simulink model "TestMotorSystem"  (R2018a)
settings: Solver=ode14x  StartTime=0.0  StopTime=10  FixedStep=Ts  RelTol=1e-3
values from neighbouring files (symbols this model uses):
  idrv = zeros(size(omegarv))    [setupTestMotorSystem.m]
  K_i = Omega_bw*R    (= 23)    [setupTestMotorSystem.m]
  K_p = Omega_bw*L    (= 0.1)    [setupTestMotorSystem.m]
  L_M = L    (= 0.001)    [setupTestMotorSystem.m]
  LamPM_M = Lambda_PM    (= 0.3)    [setupTestMotorSystem.m]
  NPoles_M = N_p    (= 6)    [setupTestMotorSystem.m]
  omegarv = linspace(0,800,1000)    [setupTestMotorSystem.m]
  Ts = 0.001    [setupTestMotorSystem.m]
undefined symbols (not defined in the file or in its folder): SJac_Per_I, Vdc_M
libraries: simulink_extras x3, simulink x2, Lib_PFSys_HiFiPMSM_TMATS x1
settings Model: Creator=glthoma1  LastModifiedBy=mebell
settings CodeAppCC: StateflowObjectComments=on

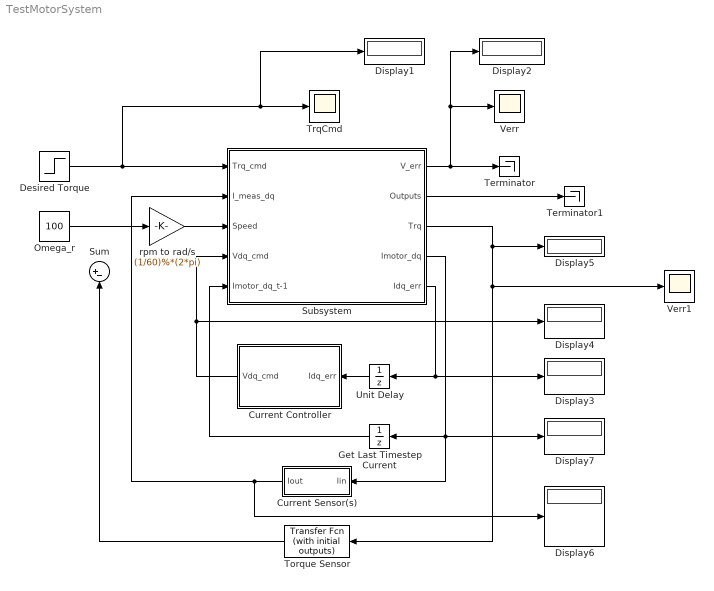
== system TestMotorSystem ==
  Current Controller : Subsystem
  Current Sensor(s) : Subsystem
  Desired Torque : Step  Time=5  Before=450  After=0  SampleTime=0
  Display{1..7} (7 alike) : Display
  Get Last Timestep Current : UnitDelay  InitialCondition=[-300; 330]  SampleTime=-1
  Omega_r : Constant  Value=100
  Subsystem : Subsystem
  Sum : Sum  Inputs=|+-
  Terminator : Terminator
  Terminator1 : Terminator
  Torque Sensor : simulink_extras/Additional Linear/Transfer Fcn (with initial outputs)  N=[10]  D="[1  10]"  Y0=450  U0=450
  TrqCmd : Scope
  Unit Delay : UnitDelay  InitialCondition=[0; 0]  SampleTime=-1
  Verr : Scope
  Verr1 : Scope
  rpm to rad/s : Gain  Gain=(1/60)%*(2*pi)
  wires:
  Desired Torque/1 -> Subsystem/1(Trq_cmd), Display1/1, TrqCmd/1
  Torque Sensor/1 -> Sum/2
  Subsystem/1(V_err) -> Terminator/1, Verr/1, Display2/1
  Current Sensor(s)/1(Iout) -> Display6/1, Subsystem/2(I_meas_dq)
  Omega_r/1 -> rpm to rad/s/1
  Subsystem/2(Outputs) -> Terminator1/1
  Subsystem/3(Trq) -> Verr1/1, Torque Sensor/1, Display5/1
  Subsystem/4(Imotor_dq) -> Current Sensor(s)/1(Iin), Display7/1, Get Last Timestep Current/1
  Subsystem/5(Idq_err) -> Display3/1, Unit Delay/1
  Current Controller/1(Vdq_cmd) -> Display4/1, Subsystem/4(Vdq_cmd)
  Unit Delay/1 -> Current Controller/1(Idq_err)
  rpm to rad/s/1 -> Subsystem/3(Speed)
  Get Last Timestep Current/1 -> Subsystem/5(Imotor_dq_t-1)

== system TestMotorSystem/Current Controller ==
  Idq_err : Inport
  Demux : Demux  Outputs=2
  Direct PID Controller : simulink/Continuous/PID Controller  Controller=PID  TimeDomain=Continuous-time  SampleTime=-1  IntegratorMethod=Forward Euler  FilterMethod=Forward Euler  Form=Parallel  UseFilter=on  ControllerParametersSource=internal  P=K_p  I=K_i  D=0  N=100  InitialConditionSource=internal  InitialConditionForIntegrator=-165  InitialConditionForFilter=0  ExternalReset=none  LimitOutput=off  UpperSaturationLimit=inf  LowerSaturationLimit=-inf  LinearizeAsGain=on  AntiWindupMode=none  Kb=1  TrackingMode=off  Kt=1  PParamMin=[]  PParamMax=[]  IParamMin=[]  IParamMax=[]  DParamMin=[]  DParamMax=[]  NParamMin=[]  NParamMax=[]  KbParamMin=[]  KbParamMax=[]  KtParamMin=[]  KtParamMax=[]  POutMin=[]  POutMax=[]  IOutMin=[]  IOutMax=[]  DOutMin=[]  DOutMax=[]  NOutMin=[]  NOutMax=[]  KbOutMin=[]  KbOutMax=[]  KtOutMin=[]  KtOutMax=[]  IntegratorOutMin=[]  IntegratorOutMax=[]  FilterOutMin=[]  FilterOutMax=[]  SumOutMin=[]  SumOutMax=[]  SumI1OutMin=[]  SumI1OutMax=[]  SumI2OutMin=[]  SumI2OutMax=[]  SumI3OutMin=[]  SumI3OutMax=[]  SumDOutMin=[]  SumDOutMax=[]  SaturationOutMin=[]  SaturationOutMax=[]  IntegratorContinuousStateAttributes=''  IntegratorStateMustResolveToSignalObject=off  IntegratorRTWStateStorageClass=Auto  FilterContinuousStateAttributes=''  FilterStateMustResolveToSignalObject=off  FilterRTWStateStorageClass=Auto  DifferentiatorICPrevScaledInput=0  DifferentiatorOutMin=[]  DifferentiatorOutMax=[]  InitialConditionSetting=State (most efficient)  FilterDiffOutCoefMin=[]  FilterDiffOutCoefMax=[]  SumDenOutMin=[]  SumDenOutMax=[]  SumNumOutMin=[]  SumNumOutMax=[]  ReciprocalOutMin=[]  ReciprocalOutMax=[]  DivideOutMin=[]  DivideOutMax=[]  TunerSelectOption=Transfer Function Based (PID Tuner App)
  Mux : Mux  Inputs=2
  Quadrature PID Controller : simulink/Continuous/PID Controller  Controller=PID  TimeDomain=Continuous-time  SampleTime=-1  IntegratorMethod=Forward Euler  FilterMethod=Forward Euler  Form=Parallel  UseFilter=on  ControllerParametersSource=internal  P=K_p  I=K_i  D=0  N=100  InitialConditionSource=internal  InitialConditionForIntegrator=76  InitialConditionForFilter=0  ExternalReset=none  LimitOutput=off  UpperSaturationLimit=inf  LowerSaturationLimit=-inf  LinearizeAsGain=on  AntiWindupMode=none  Kb=1  TrackingMode=off  Kt=1  PParamMin=[]  PParamMax=[]  IParamMin=[]  IParamMax=[]  DParamMin=[]  DParamMax=[]  NParamMin=[]  NParamMax=[]  KbParamMin=[]  KbParamMax=[]  KtParamMin=[]  KtParamMax=[]  POutMin=[]  POutMax=[]  IOutMin=[]  IOutMax=[]  DOutMin=[]  DOutMax=[]  NOutMin=[]  NOutMax=[]  KbOutMin=[]  KbOutMax=[]  KtOutMin=[]  KtOutMax=[]  IntegratorOutMin=[]  IntegratorOutMax=[]  FilterOutMin=[]  FilterOutMax=[]  SumOutMin=[]  SumOutMax=[]  SumI1OutMin=[]  SumI1OutMax=[]  SumI2OutMin=[]  SumI2OutMax=[]  SumI3OutMin=[]  SumI3OutMax=[]  SumDOutMin=[]  SumDOutMax=[]  SaturationOutMin=[]  SaturationOutMax=[]  IntegratorContinuousStateAttributes=''  IntegratorStateMustResolveToSignalObject=off  IntegratorRTWStateStorageClass=Auto  FilterContinuousStateAttributes=''  FilterStateMustResolveToSignalObject=off  FilterRTWStateStorageClass=Auto  DifferentiatorICPrevScaledInput=0  DifferentiatorOutMin=[]  DifferentiatorOutMax=[]  InitialConditionSetting=State (most efficient)  FilterDiffOutCoefMin=[]  FilterDiffOutCoefMax=[]  SumDenOutMin=[]  SumDenOutMax=[]  SumNumOutMin=[]  SumNumOutMax=[]  ReciprocalOutMin=[]  ReciprocalOutMax=[]  DivideOutMin=[]  DivideOutMax=[]  TunerSelectOption=Transfer Function Based (PID Tuner App)
  Vdq_cmd : Outport
  wires:
  Demux/2 -> Quadrature PID Controller/1
  Demux/1 -> Direct PID Controller/1
  Direct PID Controller/1 -> Mux/1
  Quadrature PID Controller/1 -> Mux/2
  Idq_err/1 -> Demux/1
  Mux/1 -> Vdq_cmd/1

== system TestMotorSystem/Current Sensor(s) ==
  Iin : Inport
  Current Sensor : simulink_extras/Additional Linear/Transfer Fcn (with initial outputs)  N=[10000]  D="[1  10000]"  Y0=-300  U0=-300
  Current Sensor1 : simulink_extras/Additional Linear/Transfer Fcn (with initial outputs)  N=[10000]  D="[1  10000]"  Y0=330  U0=330
  Demux : Demux  Outputs=2
  Mux : Mux  Inputs=2
  Iout : Outport
  wires:
  Iin/1 -> Demux/1
  Demux/1 -> Current Sensor/1
  Demux/2 -> Current Sensor1/1
  Current Sensor/1 -> Mux/1
  Current Sensor1/1 -> Mux/2
  Mux/1 -> Iout/1

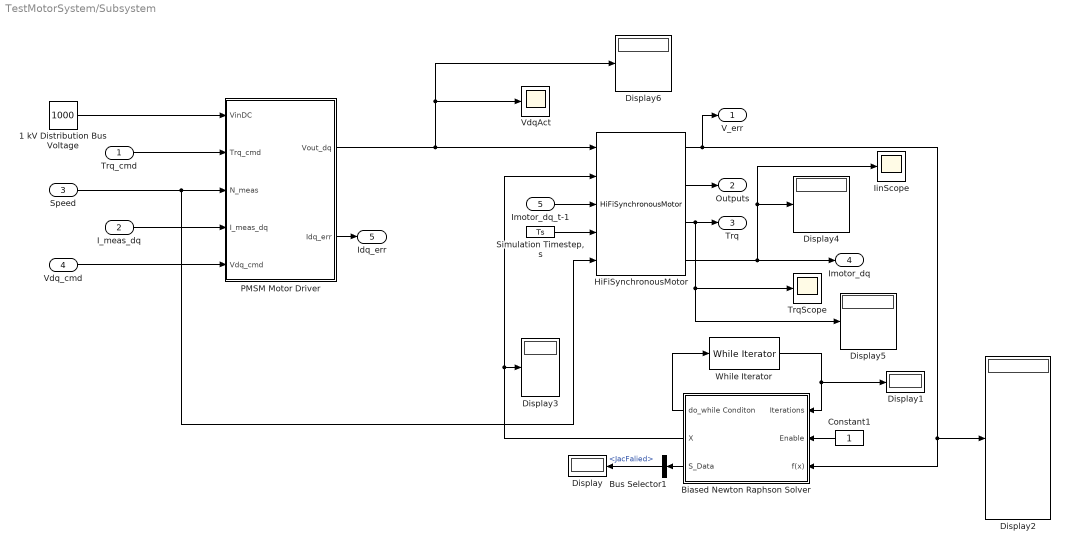
== system TestMotorSystem/Subsystem ==
  Trq_cmd : Inport
  I_meas_dq : Inport  Port=2
  Speed : Inport  Port=3
  Vdq_cmd : Inport  Port=4
  Imotor_dq_t-1 : Inport  Port=5
  1 kV Distribution Bus Voltage : Constant  Value=1000
  Biased Newton Raphson Solver : Subsystem  mask(Newton Raphson Solver){SJac_Per_M=0.001*[1; -1]*([1 1]), SNR_IC_M=[-300; 330], Shift_M=1000, SNR_DX_M=0.5, SNR_Mx_M=1e5, SNR_Mn_M=-1e5, SJacobianAttempts_M=2, Cond_Limits_M=0.001}
      mask prompts: SJac_Per_M "SJac_Per_M - Jacobian Perturbation size (frac) (nxm)"; SNR_IC_M "SNR_IC_M - Newton Raphson Initial Conditions (mx1)"; Shift_M "Shift_M - Bias to shift the solution to avoid convergence issues"; SNR_DX_M "SNR_DX_M - Newton Raphson step size limiter (%) (1x1)"; SNR_Mx_M "SNR_Mx_M - Newton Raphson max limit (1x1 or mx1)"; SNR_Mn_M "SNR_Mn_M - Newton Raphson min limit (1x1 or mx1)"; SJacobianAttempts_M "SJacobianAttempts_M - Newton Raphson attempts before the Jacobian recalculation (1x1)"; Cond_Limits_M "Cond_Limits_M - Iteration Conditions Limits (mx1 or 1x1)"
      mask help:
      | The Iterative Newton Raphson Solver with Jacobian Calculator block will
      | supply the inputs to iteratively drive the outputs of a system to zero.
      |
      | This will be performed in three steps.
      | 1) Jabobian calculator sends Perturbations to the plant then calculates the plant
      | Jacboian based on the system response
      | 2) The Newton Raphson will use the inverse of the Jacobian to iteratively step the
      | system toward solution.
      | 3) Once the solution has satisfied the conditions the Newton Raphson is shut off.
      |
      | This module is designed for dynamic systems and should be paired with
      | a "do... while" block in Simulink. The "do...while" block and this module
      | should both be located in the same subsystem as the plant that is to be solved for.
      mask init:
      | if isequal(size(SNR_Mx_M),size(SNR_IC_M))
      | elseif isequal(size(SNR_Mx_M),[1 1])
      | else
      |     disp('NR_Mx_Lim_M must be the same size as NR_IC_M or a constant')
      | end
      | 
      | if isequal(size(SNR_Mn_M),size(SNR_IC_M))
      | elseif isequal(size(SNR_Mn_M),[1 1])
      | else
      |     disp('NR_Mn_Lim_M must be the same size as NR_IC_M or a constant')
      | end
      | 
      | for i = 1:size(SJac_Per_M,1)
      |     SJac_Per_I(i,:) = SJac_Per_M(i,:).*(SNR_IC_M'./(SNR_IC_M' + Shift_M));
      | end
      mask Help: web(which('Solver_TMATS_INRSwJC.html'),'-helpbrowser')
  Bus Selector1 : BusSelector  OutputSignals=JacFalied
  Constant1 : Constant
  Display{,1..6} (7 alike) : Display
  HiFiSynchronousMotor : Lib_PFSys_HiFiPMSM_TMATS/HiFiSynchronousMotor  X_C_TorqueVec_M=[0 1000 10000]  Y_C_SpeedVec_M=[0 500 5000]  T_C_EffArray_M=[0.5 0.5 0.5; 0.5 1 1; 0.5 1 1]  R_M=R  L_M=L  LamPM_M=Lambda_PM  NPoles_M=N_p  NPhases_M=N_phases
  IinScope : Scope
  PMSM Motor Driver : Subsystem
  "Simulation Timestep, s" : Constant  Value=Ts
  TrqScope : Scope
  VdqAct : Scope
  While Iterator : WhileIterator  MaxIters=20  WhileBlockType=do-while  ShowIterationPort=on
  V_err : Outport
  Outputs : Outport  Port=2
  Trq : Outport  Port=3
  Imotor_dq : Outport  Port=4
  Idq_err : Outport  Port=5
  wires:
  HiFiSynchronousMotor/4 -> IinScope/1, Display4/1, Imotor_dq/1
  "Simulation Timestep, s"/1 -> HiFiSynchronousMotor/4
  Speed/1 -> HiFiSynchronousMotor/5, PMSM Motor Driver/3(N_meas)
  HiFiSynchronousMotor/2 -> Outputs/1
  Biased Newton Raphson Solver/2(X) -> HiFiSynchronousMotor/2, Display3/1
  Biased Newton Raphson Solver/3(S_Data) -> Bus Selector1/1
  HiFiSynchronousMotor/1 -> Display2/1, Biased Newton Raphson Solver/3(f(x)), V_err/1
  While Iterator/1 -> Biased Newton Raphson Solver/1(Iterations), Display1/1
  Biased Newton Raphson Solver/1(do_while Conditon) -> While Iterator/1
  Bus Selector1/1 -> Display/1  "<JacFalied>"
  Constant1/1 -> Biased Newton Raphson Solver/2(Enable)
  HiFiSynchronousMotor/3 -> TrqScope/1, Display5/1, Trq/1
  PMSM Motor Driver/1(Vout_dq) -> HiFiSynchronousMotor/1, Display6/1, VdqAct/1
  1 kV Distribution Bus Voltage/1 -> PMSM Motor Driver/1(VinDC)
  Trq_cmd/1 -> PMSM Motor Driver/2(Trq_cmd)
  I_meas_dq/1 -> PMSM Motor Driver/4(I_meas_dq)
  Vdq_cmd/1 -> PMSM Motor Driver/5(Vdq_cmd)
  PMSM Motor Driver/2(Idq_err) -> Idq_err/1
  Imotor_dq_t-1/1 -> HiFiSynchronousMotor/3

== system TestMotorSystem/Subsystem/Biased Newton Raphson Solver ==
  Iterations : Inport
  Enable : Inport  Port=2
  f(x) : Inport  Port=3
  Constant2 : Constant  Value=Shift_M
  Iterative NR Solver w JacobianCalc : Subsystem  mask(T-MATS: Iterative NR Solver w Jacobian Calc Library Block){SJac_Per_M=SJac_Per_I, SNR_IC_M=SNR_IC_M + Shift_M, SNR_DX_M=SNR_DX_M, SNR_Mx_M=SNR_Mx_M, SNR_Mn_M=SNR_Mn_M, SJacobianAttempts_M=SJacobianAttempts_M, Cond_Limits_M=Cond_Limits_M}
      mask prompts: SJac_Per_M "SJac_Per_M - Jacobian Perturbation size (frac) (nxm)"; SNR_IC_M "SNR_IC_M - Newton Raphson Initial Conditions (mx1)"; SNR_DX_M "SNR_DX_M - Newton Raphson step size limiter (%) (1x1)"; SNR_Mx_M "SNR_Mx_M - Newton Raphson max limit (1x1 or mx1)"; SNR_Mn_M "SNR_Mn_M - Newton Raphson min limit (1x1 or mx1)"; SJacobianAttempts_M "SJacobianAttempts_M - Newton Raphson attempts before the Jacobian recalculation (1x1)"; Cond_Limits_M "Cond_Limits_M - Iteration Conditions Limits (mx1 or 1x1)"
      mask help:
      | The Iterative Newton Raphson Solver with Jacobian Calculator block will
      | supply the inputs to iteratively drive the outputs of a system to zero.
      |
      | This will be performed in three steps.
      | 1) Jabobian calculator sends Perturbations to the plant then calculates the plant
      | Jacboian based on the system response
      | 2) The Newton Raphson will use the inverse of the Jacobian to iteratively step the
      | system toward solution.
      | 3) Once the solution has satisfied the conditions the Newton Raphson is shut off.
      |
      | This module is designed for dynamic systems and should be paired with
      | a "do... while" block in Simulink. The "do...while" block and this module
      | should both be located in the same subsystem as the plant that is to be solved for.
      mask init:
      | if isequal(size(SNR_Mx_M),size(SNR_IC_M))
      | elseif isequal(size(SNR_Mx_M),[1 1])
      | else
      |     disp('NR_Mx_Lim_M must be the same size as NR_IC_M or a constant')
      | end
      | 
      | if isequal(size(SNR_Mn_M),size(SNR_IC_M))
      | elseif isequal(size(SNR_Mn_M),[1 1])
      | else
      |     disp('NR_Mn_Lim_M must be the same size as NR_IC_M or a constant')
      | end
      mask Help: web(which('Solver_TMATS_INRSwJC.html'),'-helpbrowser')
  Sum : Sum  Inputs=|+-
  do_while Conditon : Outport
  X : Outport  Port=2
  S_Data : Outport  Port=3
  wires:
  Constant2/1 -> Sum/2
  Iterative NR Solver w JacobianCalc/2(X) -> Sum/1
  f(x)/1 -> Iterative NR Solver w JacobianCalc/3(f(x))
  Iterations/1 -> Iterative NR Solver w JacobianCalc/1(Iterations)
  Enable/1 -> Iterative NR Solver w JacobianCalc/2(Enable)
  Iterative NR Solver w JacobianCalc/3(S_Data) -> S_Data/1
  Iterative NR Solver w JacobianCalc/1(do_while Condition) -> do_while Conditon/1
  Sum/1 -> X/1

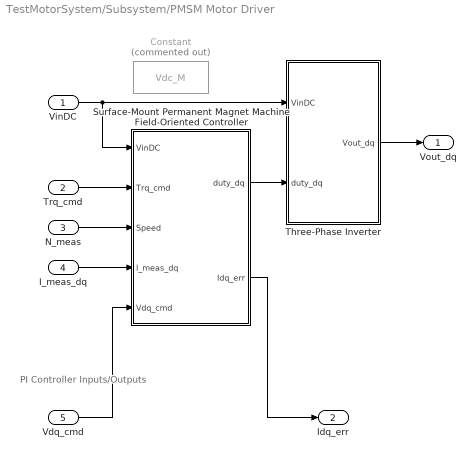
== system TestMotorSystem/Subsystem/PMSM Motor Driver ==
  note: PI Controller
      | Inputs/Outputs
  VinDC : Inport
  Trq_cmd : Inport  Port=2
  N_meas : Inport  Port=3
  I_meas_dq : Inport  Port=4
  Vdq_cmd : Inport  Port=5
  Constant : Constant  Commented=on  Value=Vdc_M
  Surface-Mount Permanent Magnet Machine Field-Oriented Controller : Subsystem
  Three-Phase Inverter : Subsystem
  Vout_dq : Outport
  Idq_err : Outport  Port=2
  wires:
  N_meas/1 -> Surface-Mount Permanent Magnet Machine Field-Oriented Controller/3(Speed)
  Surface-Mount Permanent Magnet Machine Field-Oriented Controller/1(duty_dq) -> Three-Phase Inverter/2(duty_dq)
  Trq_cmd/1 -> Surface-Mount Permanent Magnet Machine Field-Oriented Controller/2(Trq_cmd)
  I_meas_dq/1 -> Surface-Mount Permanent Magnet Machine Field-Oriented Controller/4(I_meas_dq)
  Three-Phase Inverter/1(Vout_dq) -> Vout_dq/1
  Surface-Mount Permanent Magnet Machine Field-Oriented Controller/2(Idq_err) -> Idq_err/1
  Vdq_cmd/1 -> Surface-Mount Permanent Magnet Machine Field-Oriented Controller/5(Vdq_cmd)
  VinDC/1 -> Surface-Mount Permanent Magnet Machine Field-Oriented Controller/1(VinDC), Three-Phase Inverter/1(VinDC)

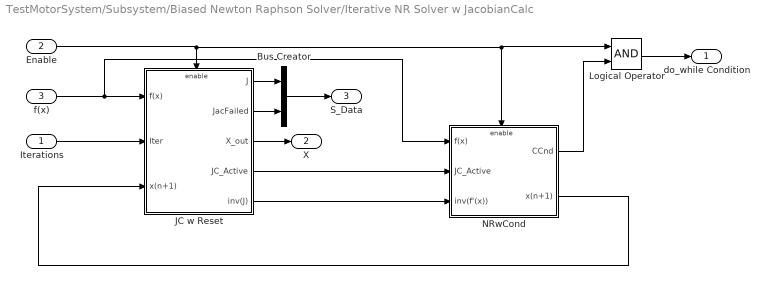
== system TestMotorSystem/Subsystem/Biased Newton Raphson Solver/Iterative NR Solver w JacobianCalc ==
  Iterations : Inport  PortDimensions=1
  Enable : Inport  Port=2  PortDimensions=1
  f(x) : Inport  Port=3  PortDimensions=length(SNR_IC_M)
  Bus Creator : BusCreator  Inputs=2
  JC w Reset : Subsystem
  Logical Operator : Logic  AllPortsSameDT=off  OutDataTypeStr=boolean
  NRwCond : Subsystem
  do_while Condition : Outport  PortDimensions=1
  X : Outport  Port=2  PortDimensions=length(SNR_IC_M)
  S_Data : Outport  Port=3
  wires:
  f(x)/1 -> NRwCond/1(f(x)), JC w Reset/1(f(x))
  NRwCond/1(CCnd) -> Logical Operator/2
  Iterations/1 -> JC w Reset/2(Iter)
  NRwCond/2(x(n+1)) -> JC w Reset/3(x(n+1))
  JC w Reset/1(J) -> Bus Creator/1
  JC w Reset/3(X_out) -> X/1
  JC w Reset/4(JC_Active) -> NRwCond/2(JC_Active)
  JC w Reset/5(inv(J)) -> NRwCond/3(inv(f'(x)))
  Enable/1 -> JC w Reset/Enable, NRwCond/Enable, Logical Operator/1
  Logical Operator/1 -> do_while Condition/1
  Bus Creator/1 -> S_Data/1
  JC w Reset/2(JacFailed) -> Bus Creator/2

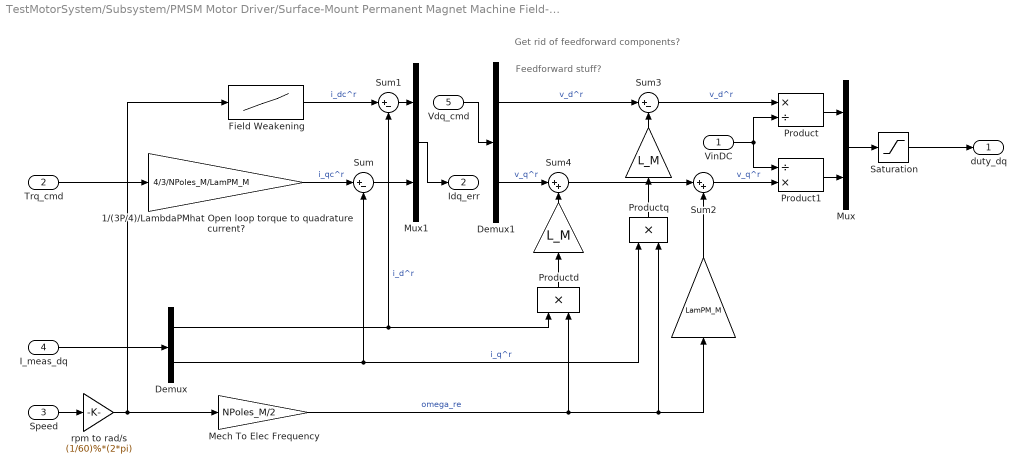
== system TestMotorSystem/Subsystem/PMSM Motor Driver/Surface-Mount Permanent Magnet Machine Field-Oriented Controller ==
  note: Feedforward stuff?
  note: Get rid of feedforward components?
  VinDC : Inport
  Trq_cmd : Inport  Port=2
  Speed : Inport  Port=3
  I_meas_dq : Inport  Port=4
  Vdq_cmd : Inport  Port=5
  "  " : Gain  Gain=L_M  SaturateOnIntegerOverflow=on  OutDataTypeStr=Inherit: Same as input  ParamDataTypeStr=Inherit: Same as input
  "   " : Gain  Gain=LamPM_M  SaturateOnIntegerOverflow=on  OutDataTypeStr=Inherit: Same as input  ParamDataTypeStr=Inherit: Same as input
  "      " : Gain  Gain=L_M  SaturateOnIntegerOverflow=on  OutDataTypeStr=Inherit: Same as input  ParamDataTypeStr=Inherit: Same as input
  1/(3P/4)/LambdaPMhat Open loop torque to quadrature current? : Gain  Gain=4/3/NPoles_M/LamPM_M  SaturateOnIntegerOverflow=on  OutDataTypeStr=Inherit: Same as input  ParamDataTypeStr=Inherit: Same as input
  Demux : Demux  Outputs=2
  Demux1 : Demux  Outputs=2
  Field Weakening : Lookup_n-D  NumberOfTableDimensions=1  BreakpointsForDimension1=omegarv  Table=idrv  InternalRulePriority=Speed  RndMeth=Simplest  InputSameDT=on
  Mech To Elec Frequency : Gain  Gain=NPoles_M/2  SaturateOnIntegerOverflow=on  OutDataTypeStr=Inherit: Same as input  ParamDataTypeStr=Inherit: Same as input
  Mux : Mux  Inputs=2
  Mux1 : Mux  Inputs=2
  Product : Product  Inputs=*/  SaturateOnIntegerOverflow=on  OutDataTypeStr=Inherit: Same as first input
  Product1 : Product  Inputs=/*  SaturateOnIntegerOverflow=on  OutDataTypeStr=Inherit: Same as first input
  Productd : Product  SaturateOnIntegerOverflow=on  OutDataTypeStr=Inherit: Same as first input
  Productq : Product  SaturateOnIntegerOverflow=on  OutDataTypeStr=Inherit: Same as first input
  Saturation : Saturate  UpperLimit=1  LowerLimit=0
  Sum : Sum  Inputs=|+-  SaturateOnIntegerOverflow=on
  Sum1 : Sum  Inputs=|+-  SaturateOnIntegerOverflow=on
  Sum2 : Sum  Inputs=|++  SaturateOnIntegerOverflow=on
  Sum3 : Sum  Inputs=|+-  SaturateOnIntegerOverflow=on
  Sum4 : Sum  Inputs=|++  SaturateOnIntegerOverflow=on
  rpm to rad/s : Gain  Gain=(1/60)%*(2*pi)
  duty_dq : Outport
  Idq_err : Outport  Port=2
  wires:
  Trq_cmd/1 -> 1/(3P/4)/LambdaPMhat Open loop torque to quadrature current?/1
  1/(3P/4)/LambdaPMhat Open loop torque to quadrature current?/1 -> Sum/1  "i_qc^r"
  Demux/1 -> Productd/1, Sum1/2  "i_d^r"
  Demux/2 -> Productq/1, Sum/2  "i_q^r"
  Field Weakening/1 -> Sum1/1  "i_dc^r"
  Sum1/1 -> Mux1/1
  Sum/1 -> Mux1/2
  Mech To Elec Frequency/1 -> "   "/1, Productq/2, Productd/2  "omega_re"
  Productq/1 -> "      "/1
  Sum3/1 -> Product/1  "v_d^r"
  "      "/1 -> Sum3/2
  "  "/1 -> Sum4/2
  Productd/1 -> "  "/1
  Demux1/2 -> Sum4/1  "v_q^r"
  Sum4/1 -> Sum2/1
  "   "/1 -> Sum2/2
  I_meas_dq/1 -> Demux/1
  Vdq_cmd/1 -> Demux1/1
  Mux1/1 -> Idq_err/1
  Demux1/1 -> Sum3/1  "v_d^r"
  Sum2/1 -> Product1/2  "v_q^r"
  VinDC/1 -> Product/2, Product1/1
  Product/1 -> Mux/1
  Product1/1 -> Mux/2
  Mux/1 -> Saturation/1
  Speed/1 -> rpm to rad/s/1
  rpm to rad/s/1 -> Mech To Elec Frequency/1, Field Weakening/1
  Saturation/1 -> duty_dq/1

== system TestMotorSystem/Subsystem/PMSM Motor Driver/Three-Phase Inverter ==
  VinDC : Inport
  duty_dq : Inport  Port=2
  Product : Product
  Vout_dq : Outport
  wires:
  duty_dq/1 -> Product/2
  VinDC/1 -> Product/1
  Product/1 -> Vout_dq/1

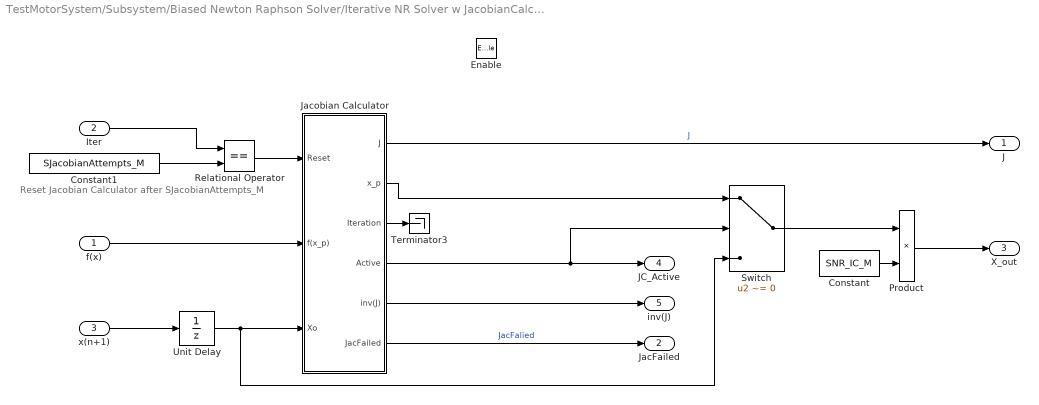
== system TestMotorSystem/Subsystem/Biased Newton Raphson Solver/Iterative NR Solver w JacobianCalc/JC w Reset ==
  note: Reset Jacobian Calculator after SJacobianAttempts_M
  f(x) : Inport  PortDimensions=length(SNR_IC_M)
  Iter : Inport  Port=2  PortDimensions=1
  x(n+1) : Inport  Port=3
  Enable : EnablePort
  Constant : Constant  Value=SNR_IC_M
  Constant1 : Constant  Value=SJacobianAttempts_M  OutDataTypeStr=uint32
  Jacobian Calculator : Subsystem  TreatAsAtomicUnit=on  mask(T-MATS: Jacobian Calculator Library Block){N_Per_M=SJac_Per_M}
      mask prompts: N_Per_M "N_Per_M - Perturbations (nxm)"
      mask help:
      | The Jacobian Calculator block calculates the Jabobian of the system by perturbing the system around an initial point and calculating the gradient for each perturbation. This module will run once on start up and then again only if the reset is pressed.
      | Below: n (rows) is the number of times each independent will be perturbed and m (columns) is the number of inputs.
      mask Help: web(which('NumMthd_TMATS_JC.html'),'-helpbrowser')
  Product : Product  RndMeth=Zero
  Relational Operator : RelationalOperator  Operator===  OutDataTypeStr=boolean  RndMeth=Nearest
  Switch : Switch  Criteria=u2 ~= 0  Threshold=1
  Terminator3 : Terminator
  Unit Delay : UnitDelay  InitialCondition=ones(length(SNR_IC_M),1)  SampleTime=-1
  J : Outport  PortDimensions=[length(SNR_IC_M),length(SNR_IC_M)]
  JacFailed : Outport  Port=2  PortDimensions=1
  X_out : Outport  Port=3  PortDimensions=length(SNR_IC_M)
  JC_Active : Outport  Port=4  PortDimensions=1
  inv(J) : Outport  Port=5  PortDimensions=[length(SNR_IC_M),length(SNR_IC_M)]
  wires:
  f(x)/1 -> Jacobian Calculator/2(f(x_p))
  Jacobian Calculator/5(inv(J)) -> inv(J)/1
  Unit Delay/1 -> Switch/3, Jacobian Calculator/3(Xo)
  x(n+1)/1 -> Unit Delay/1
  Jacobian Calculator/1(J) -> J/1  "J"
  Constant/1 -> Product/2
  Relational Operator/1 -> Jacobian Calculator/1(Reset)
  Product/1 -> X_out/1
  Jacobian Calculator/2(x_p) -> Switch/1
  Switch/1 -> Product/1
  Jacobian Calculator/4(Active) -> Switch/2, JC_Active/1
  Constant1/1 -> Relational Operator/2
  Iter/1 -> Relational Operator/1
  Jacobian Calculator/3(Iteration) -> Terminator3/1
  Jacobian Calculator/6(JacFailed) -> JacFailed/1  "JacFalied"

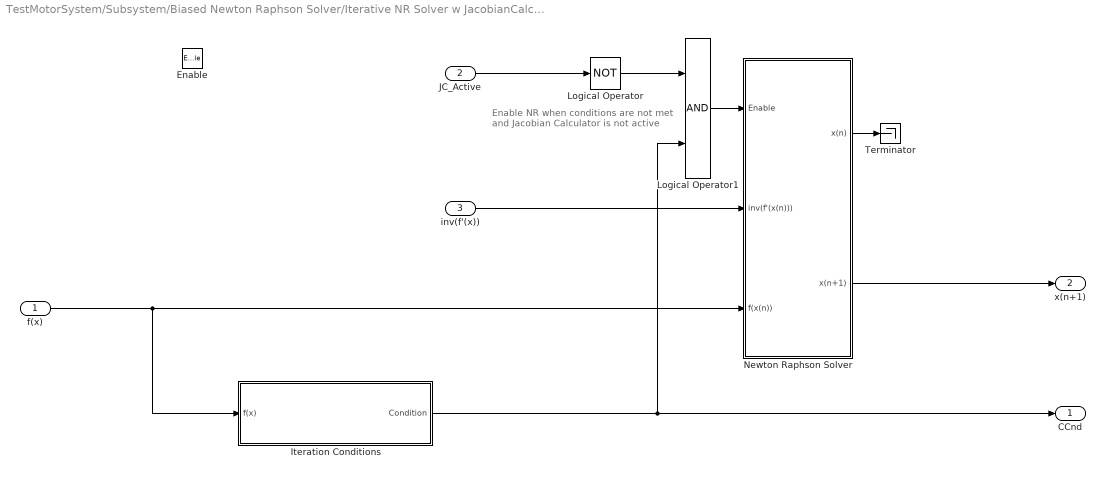
== system TestMotorSystem/Subsystem/Biased Newton Raphson Solver/Iterative NR Solver w JacobianCalc/NRwCond ==
  note: Enable NR when conditions are not met
      | and Jacobian Calculator is not active
  f(x) : Inport  PortDimensions=length(SNR_IC_M)
  JC_Active : Inport  Port=2  PortDimensions=1
  inv(f'(x)) : Inport  Port=3  PortDimensions=[length(SNR_IC_M),length(SNR_IC_M)]
  Enable : EnablePort
  Iteration Conditions : Subsystem
  Logical Operator : Logic  Operator=NOT  AllPortsSameDT=off  OutDataTypeStr=boolean
  Logical Operator1 : Logic  AllPortsSameDT=off  OutDataTypeStr=boolean
  Newton Raphson Solver : Subsystem  TreatAsAtomicUnit=on  mask(T-MATS: Newton Raphson Solver Library Block){NR_IC_M=ones(size(SNR_IC_M)), NR_dx_Lim_M=SNR_DX_M, NR_Mx_Lim_M=SNR_Mx_M./SNR_IC_M, NR_Mn_Lim_M=SNR_Mn_M./SNR_IC_M, BlkNm_M=double(gcb)}
      mask prompts: NR_IC_M "NR_IC_M - Initial Conditions of Newton Raphson (mx1)"; NR_dx_Lim_M "NR_dx_Lim_M - Newton Raphson step size limit (%) (1x1)"; NR_Mx_Lim_M "NR_Mx_Lim_M - Max limit (1x1 or mx1)"; NR_Mn_Lim_M "NR_Mn_Lim_M - Min Limit (1x1 or mx1)"; BlkNm_M "BlkNm_M - Block Name"
      mask help:
      | Newton Raphson Solver:
      |
      | x(n+1) = x(n) - inverse(f'(x(n)))*f(x(n))
      |
      | Note:
      | inverse(f'(x(n))) is an m x m matrix and f(x(n)) is an m x 1 matrix
      | where m is the length of the initial conditions matrix and number of system independents.
      mask init:
      | if isequal(size(NR_Mx_Lim_M),size(NR_IC_M))
      | elseif isequal(size(NR_Mx_Lim_M),size(1))
      | else
      |     warning('NR_Mx_Lim_M must be the same size as NR_IC_M or a constant')
      | end
      | 
      | if isequal(size(NR_Mn_Lim_M),size(NR_IC_M))
      | elseif isequal(size(NR_Mn_Lim_M),size(1))
      | else
      |     warning('NR_Mn_Lim_M must be the same size as NR_IC_M or a constant')
      | end
      mask Help: web(which('NumMthd_TMATS_NRS.html'),'-helpbrowser')
  Terminator : Terminator
  CCnd : Outport  PortDimensions=1
  x(n+1) : Outport  Port=2  PortDimensions=length(SNR_IC_M)
  wires:
  f(x)/1 -> Iteration Conditions/1(f(x)), Newton Raphson Solver/3(f(x(n)))
  JC_Active/1 -> Logical Operator/1
  Newton Raphson Solver/2(x(n+1)) -> x(n+1)/1
  Newton Raphson Solver/1(x(n)) -> Terminator/1
  inv(f'(x))/1 -> Newton Raphson Solver/2(inv(f'(x(n))))
  Logical Operator1/1 -> Newton Raphson Solver/1(Enable)
  Logical Operator/1 -> Logical Operator1/1
  Iteration Conditions/1(Condition) -> Logical Operator1/2, CCnd/1

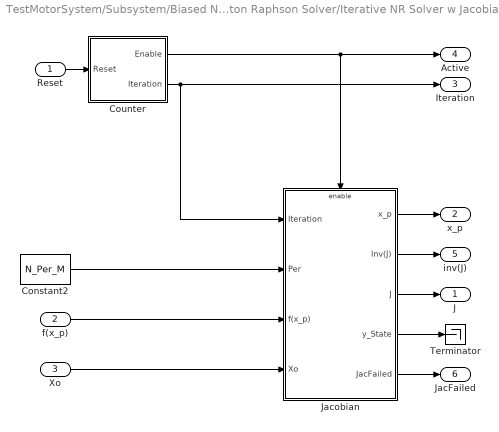
== system TestMotorSystem/Subsystem/Biased Newton Raphson Solver/Iterative NR Solver w JacobianCalc/JC w Reset/Jacobian Calculator ==
  Reset : Inport  PortDimensions=1
  f(x_p) : Inport  Port=2  PortDimensions=size(N_Per_M,2)
  Xo : Inport  Port=3  PortDimensions=size(N_Per_M,2)
  Constant2 : Constant  Value=N_Per_M
  Counter : Subsystem  mask{N_Ind_M=prod(size(N_Per_M))}
      mask prompts: N_Ind_M "number of independents, N_Ind_M"
  Jacobian : Subsystem
  Terminator : Terminator
  J : Outport  PortDimensions=[size(N_Per_M,2), size(N_Per_M,2)]
  x_p : Outport  Port=2  PortDimensions=size(N_Per_M,2)
  Iteration : Outport  Port=3  PortDimensions=1
  Active : Outport  Port=4  PortDimensions=1
  inv(J) : Outport  Port=5  PortDimensions=[size(N_Per_M,2), size(N_Per_M,2)]
  JacFailed : Outport  Port=6  PortDimensions=1
  wires:
  f(x_p)/1 -> Jacobian/3(f(x_p))
  Constant2/1 -> Jacobian/2(Per)
  Jacobian/1(x_p) -> x_p/1
  Reset/1 -> Counter/1(Reset)
  Counter/1(Enable) -> Active/1, Jacobian/Enable
  Xo/1 -> Jacobian/4(Xo)
  Counter/2(Iteration) -> Iteration/1, Jacobian/1(Iteration)
  Jacobian/2(Inv(J)) -> inv(J)/1
  Jacobian/3(J) -> J/1
  Jacobian/4(y_State) -> Terminator/1
  Jacobian/5(JacFailed) -> JacFailed/1

== system TestMotorSystem/Subsystem/Biased Newton Raphson Solver/Iterative NR Solver w JacobianCalc/NRwCond/Iteration Conditions ==
  f(x) : Inport
  Abs : Abs
  Constant1 : Constant  Value=Cond_Limits_M
  Constant2 : Constant  Value=0
  Relational Operator : RelationalOperator  Operator=>  OutDataTypeStr=boolean  RndMeth=Nearest
  Relational Operator1 : RelationalOperator  Operator=>  OutDataTypeStr=boolean  RndMeth=Nearest
  Sum of Elements : Sum  Inputs=+
  Condition : Outport
  wires:
  Relational Operator1/1 -> Condition/1
  Sum of Elements/1 -> Relational Operator1/1
  Constant2/1 -> Relational Operator1/2
  Relational Operator/1 -> Sum of Elements/1
  f(x)/1 -> Abs/1
  Constant1/1 -> Relational Operator/2
  Abs/1 -> Relational Operator/1

== system TestMotorSystem/Subsystem/Biased Newton Raphson Solver/Iterative NR Solver w JacobianCalc/NRwCond/Newton Raphson Solver ==
  Enable : Inport  PortDimensions=1
  inv(f'(x(n))) : Inport  Port=2  PortDimensions=[length(NR_IC_M),length(NR_IC_M)]
  f(x(n)) : Inport  Port=3  PortDimensions=length(NR_IC_M)
  NR Update : Subsystem
  Switch : Switch  Criteria=u2 > Threshold
  Unit Delay : UnitDelay  InitialCondition=NR_IC_M  SampleTime=-1
  x(n) : Outport  PortDimensions=length(NR_IC_M)
  x(n+1) : Outport  Port=2  PortDimensions=length(NR_IC_M)
  wires:
  Unit Delay/1 -> x(n)/1, Switch/3, NR Update/3(x(n))
  Enable/1 -> Switch/2, NR Update/Enable
  Switch/1 -> Unit Delay/1, x(n+1)/1
  f(x(n))/1 -> NR Update/1(f(x))
  inv(f'(x(n)))/1 -> NR Update/2(inv(J))
  NR Update/1(x(n+1)) -> Switch/1

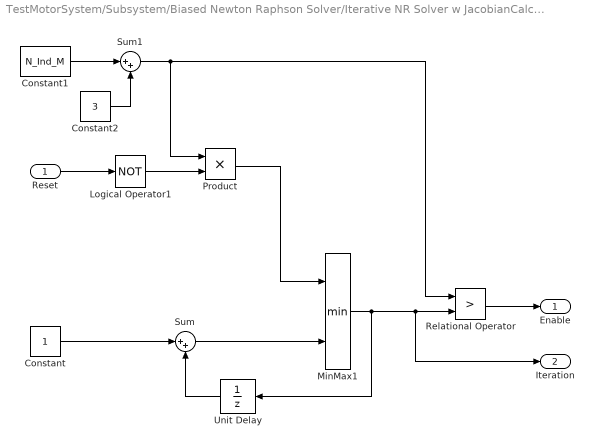
== system TestMotorSystem/Subsystem/Biased Newton Raphson Solver/Iterative NR Solver w JacobianCalc/JC w Reset/Jacobian Calculator/Counter ==
  Reset : Inport
  Constant : Constant
  Constant1 : Constant  Value=N_Ind_M
  Constant2 : Constant  Value=3
  Logical Operator1 : Logic  Operator=NOT  AllPortsSameDT=off  OutDataTypeStr=boolean
  MinMax1 : MinMax  Inputs=2
  Product : Product  RndMeth=Zero
  Relational Operator : RelationalOperator  Operator=>  OutDataTypeStr=boolean  RndMeth=Nearest
  Sum : Sum  Inputs=|++
  Sum1 : Sum  Inputs=|++
  Unit Delay : UnitDelay  SampleTime=-1
  Enable : Outport
  Iteration : Outport  Port=2
  wires:
  Constant/1 -> Sum/1
  Product/1 -> MinMax1/1
  Sum/1 -> MinMax1/2
  Unit Delay/1 -> Sum/2
  MinMax1/1 -> Unit Delay/1, Iteration/1, Relational Operator/2
  Relational Operator/1 -> Enable/1
  Logical Operator1/1 -> Product/2
  Reset/1 -> Logical Operator1/1
  Sum1/1 -> Relational Operator/1, Product/1
  Constant2/1 -> Sum1/2
  Constant1/1 -> Sum1/1

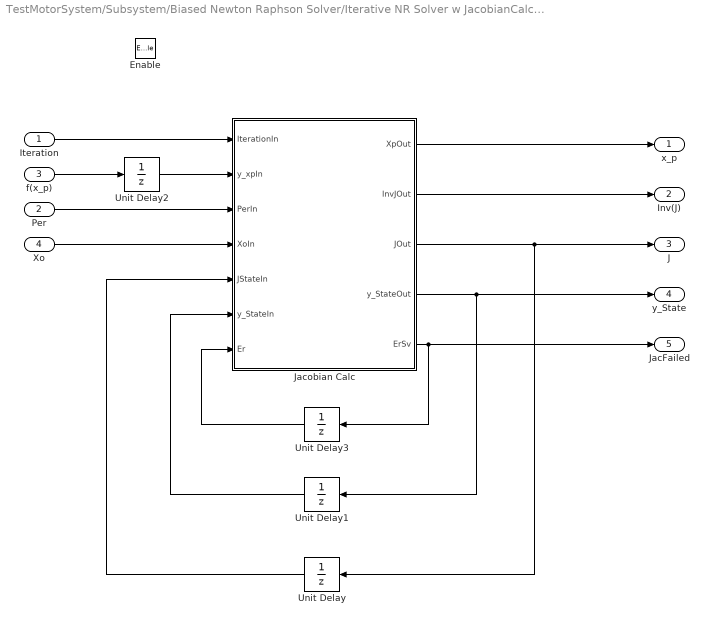
== system TestMotorSystem/Subsystem/Biased Newton Raphson Solver/Iterative NR Solver w JacobianCalc/JC w Reset/Jacobian Calculator/Jacobian ==
  Iteration : Inport
  Per : Inport  Port=2
  f(x_p) : Inport  Port=3
  Xo : Inport  Port=4
  Enable : EnablePort
  Jacobian Calc : MATLAB Function  TreatAsAtomicUnit=on
  Unit Delay : UnitDelay  InitialCondition=zeros(size(N_Per_M,2),size(N_Per_M,2))  SampleTime=-1
  Unit Delay1 : UnitDelay  InitialCondition=zeros(size(N_Per_M,2),prod(size(N_Per_M))+1)  SampleTime=-1
  Unit Delay2 : UnitDelay  InitialCondition=zeros(size(N_Per_M,2),1)  SampleTime=-1
  Unit Delay3 : UnitDelay  SampleTime=-1
  x_p : Outport
  Inv(J) : Outport  Port=2
  J : Outport  Port=3
  y_State : Outport  Port=4
  JacFailed : Outport  Port=5
  wires:
  Jacobian Calc/1(XpOut) -> x_p/1
  Xo/1 -> Jacobian Calc/4(XoIn)
  Per/1 -> Jacobian Calc/3(PerIn)
  Iteration/1 -> Jacobian Calc/1(IterationIn)
  Jacobian Calc/3(JOut) -> Unit Delay/1, J/1
  Jacobian Calc/2(InvJOut) -> Inv(J)/1
  Unit Delay/1 -> Jacobian Calc/5(JStateIn)
  Jacobian Calc/4(y_StateOut) -> Unit Delay1/1, y_State/1
  Unit Delay1/1 -> Jacobian Calc/6(y_StateIn)
  f(x_p)/1 -> Unit Delay2/1
  Unit Delay2/1 -> Jacobian Calc/2(y_xpIn)
  Jacobian Calc/5(ErSv) -> Unit Delay3/1, JacFailed/1
  Unit Delay3/1 -> Jacobian Calc/7(Er)

== system TestMotorSystem/Subsystem/Biased Newton Raphson Solver/Iterative NR Solver w JacobianCalc/NRwCond/Newton Raphson Solver/NR Update ==
  f(x) : Inport
  inv(J) : Inport  Port=2
  x(n) : Inport  Port=3
  Enable : EnablePort
  Bounding : Subsystem
  MatrixMult : Subsystem
  Sum : Sum  Inputs=|-+
  dxLimit : Subsystem
  x(n+1) : Outport
  wires:
  f(x)/1 -> MatrixMult/1(f(x(n)))
  Sum/1 -> Bounding/1(x(n+1)raw)
  MatrixMult/1(DTS) -> dxLimit/1(dx)
  dxLimit/1(dx_limited) -> Sum/1
  inv(J)/1 -> MatrixMult/2(inv(f'(x(n))))
  Bounding/1(x(n+1)Lim) -> x(n+1)/1
  x(n)/1 -> dxLimit/2(x), Sum/2

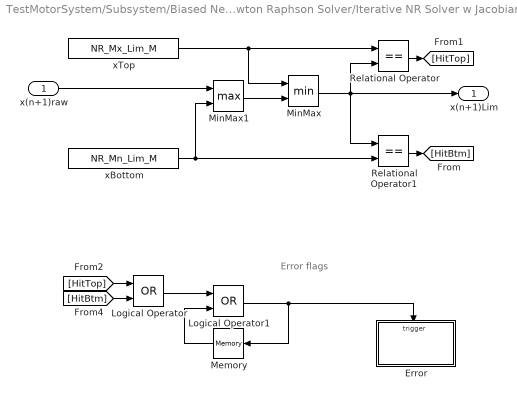
== system TestMotorSystem/Subsystem/Biased Newton Raphson Solver/Iterative NR Solver w JacobianCalc/NRwCond/Newton Raphson Solver/NR Update/Bounding ==
  note: Error flags
  x(n+1)raw : Inport
  Error : Subsystem
  Logical Operator : Logic  Operator=OR  AllPortsSameDT=off  OutDataTypeStr=boolean
  Logical Operator1 : Logic  Operator=OR  AllPortsSameDT=off  OutDataTypeStr=boolean
  Memory : Memory  InheritSampleTime=on
  MinMax : MinMax  Inputs=2
  MinMax1 : MinMax  Function=max  Inputs=2
  Relational Operator : RelationalOperator  Operator===  OutDataTypeStr=boolean  RndMeth=Nearest
  Relational Operator1 : RelationalOperator  Operator===  OutDataTypeStr=boolean  RndMeth=Nearest
  xBottom : Constant  Value=NR_Mn_Lim_M
  xTop : Constant  Value=NR_Mx_Lim_M
  x(n+1)Lim : Outport
  wires:
  xBottom/1 -> MinMax1/2, Relational Operator1/2
  x(n+1)raw/1 -> MinMax1/1
  xTop/1 -> Relational Operator/1, MinMax/1
  MinMax1/1 -> MinMax/2
  MinMax/1 -> Relational Operator1/1, Relational Operator/2, x(n+1)Lim/1
  Relational Operator1/1 -> [HitBtm]
  Relational Operator/1 -> [HitTop]
  [HitTop] -> Logical Operator/1
  Logical Operator/1 -> Logical Operator1/1
  [HitBtm] -> Logical Operator/2
  Memory/1 -> Logical Operator1/2
  Logical Operator1/1 -> Error/Trigger, Memory/1

== system TestMotorSystem/Subsystem/Biased Newton Raphson Solver/Iterative NR Solver w JacobianCalc/NRwCond/Newton Raphson Solver/NR Update/MatrixMult ==
  f(x(n)) : Inport
  inv(f'(x(n))) : Inport  Port=2
  Product : Product  Multiplication=Matrix(*)  RndMeth=Zero
  DTS : Outport
  wires:
  Product/1 -> DTS/1
  f(x(n))/1 -> Product/2
  inv(f'(x(n)))/1 -> Product/1

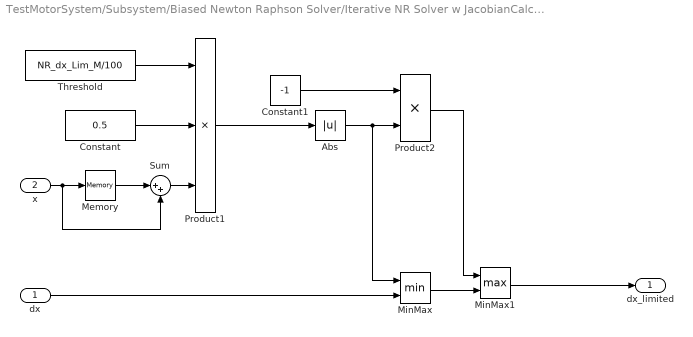
== system TestMotorSystem/Subsystem/Biased Newton Raphson Solver/Iterative NR Solver w JacobianCalc/NRwCond/Newton Raphson Solver/NR Update/dxLimit ==
  dx : Inport
  x : Inport  Port=2
  Abs : Abs
  Constant : Constant  Value=0.5
  Constant1 : Constant  Value=-1
  Memory : Memory  InitialCondition=NR_IC_M  InheritSampleTime=on
  MinMax : MinMax  Inputs=2
  MinMax1 : MinMax  Function=max  Inputs=2
  Product1 : Product  Inputs=3  RndMeth=Zero
  Product2 : Product  RndMeth=Zero
  Sum : Sum  Inputs=|++
  Threshold : Constant  Value=NR_dx_Lim_M/100
  dx_limited : Outport
  wires:
  MinMax1/1 -> dx_limited/1
  Constant1/1 -> Product2/1
  Product2/1 -> MinMax1/1
  MinMax/1 -> MinMax1/2
  dx/1 -> MinMax/2
  Abs/1 -> Product2/2, MinMax/1
  Product1/1 -> Abs/1
  Threshold/1 -> Product1/1
  x/1 -> Memory/1, Sum/2
  Constant/1 -> Product1/2
  Memory/1 -> Sum/1
  Sum/1 -> Product1/3

== system TestMotorSystem/Subsystem/Biased Newton Raphson Solver/Iterative NR Solver w JacobianCalc/NRwCond/Newton Raphson Solver/NR Update/Bounding/Error ==
  Trigger : TriggerPort  VariantControl=Variant
  MATLAB Function : MATLAB Function  TreatAsAtomicUnit=on

== matlab function TestMotorSystem/Subsystem/Biased Newton Raphson Solver/Iterative NR Solver w JacobianCalc/JC w Reset/Jacobian Calculator/Jacobian/Jacobian Calc ==
  data: IterationIn input; XpOut output; y_xpIn input; PerIn input; XoIn input; InvJOut output; JOut output; JStateIn input; y_StateIn input; y_StateOut output; Er input; ErSv output
function [XpOut, InvJOut, JOut, y_StateOut, ErSv] = fcn(IterationIn, y_xpIn, PerIn, XoIn, JStateIn, y_StateIn, Er)

% Set inital condiations
i = IterationIn;
XpOut = XoIn;
InvJOut = zeros(length(XoIn));
JOut = JStateIn;
y_StateOut = y_StateIn;
PerVec = reshape(PerIn',1,[]);
LenPV = length(PerVec);
LenXo = length(XoIn);
ErSv = Er;

% Begin taking data from f(x) at iteration a+1
a = 1;
% Begin determining Jacobian at iteration b+1
b = a+1;

% Set Xp Output
if i > a && i <= LenPV + a
    current_Xp = mod(i-a-1,LenXo)+1;
    XpOut(current_Xp) = XpOut(current_Xp) + PerVec(i - a);
end

% save state feedback
if LenXo == 1
    if i >= b;
        y_StateOut(i-a) = y_xpIn;
    end
else
    if i > a && i<= LenPV + a+1;
        y_StateOut(:,i - a) = y_xpIn;
    end
end

% Create Jacobian
if i == LenPV + b
    % Generate Jacobian matrices for each set, stacked.
    if LenXo == 1
        JMtx_extended = (y_StateOut(2:end)' - repmat(y_StateOut(1),1,LenPV))./PerVec;
    else
        JMtx_extended = (y_StateOut(:,2:end) - repmat(y_StateOut(:,1),1,LenPV))./repmat(PerVec,LenXo,1);
    end
    
    % Initialize sum matricies
    JMtrx_sum = zeros(LenXo);
    Nsum = zeros(LenXo);
    
    % determine how many perturbation sets there are, b/c MATLAB likes to
    % flip vectors when they enter MATLAB functions from Simulink for no reason.
    if min(size(PerIn)) == 1
     if LenXo == 1;
        PerNum = length(PerIn); 
     else 
        PerNum = 1;
     end
    else
        PerNum = size(PerIn,1);
    end
    
    for set = 1: PerNum
        % Break out Jacobian matrix for the current perturbation set
        JMtrx_cur = JMtx_extended(:, LenXo*(set-1)+1:LenXo*set);
        % Sum Jacobian matrices for each set
        JMtrx_sum = JMtrx_sum + JMtrx_cur(:,1:LenXo);
        % Sum number of acceptable values
        Nsum = Nsum + abs(sign(JMtrx_cur(:,1:LenXo)));
    end
    
    % Average Jacobian Matricies
    Javg = JMtrx_sum./max(Nsum,1);
    
    JOut = Javg;
    
    % Invert Jacobian
    if rank(JOut) == length(InvJOut)
        InvJOut = inv(JOut(:,:));
    elseif ErSv < 1
        disp('Jacobian can not be inverted.');
        ErSv = 1;
    end
end

== matlab function TestMotorSystem/Subsystem/Biased Newton Raphson Solver/Iterative NR Solver w JacobianCalc/NRwCond/Newton Raphson Solver/NR Update/Bounding/Error/MATLAB Function ==
  data: BlkNm_M parameter
function fcn(BlkNm_M)
%# Limit Newton Raphson outputs and produce a warning if it occurs
BName = BlkNm_M;
disp(['Warning in ' BName ': Solver limit has been hit, check for system convergence']);
